simulink library "Control_Signal_Sources"  (R2019b)
settings: Solver=VariableStepAuto  StartTime=0.0  StopTime=10.0  RelTol=1e-3
libraries: simulink x1
settings Model: Creator=mehdi  LastModifiedBy=mehdi

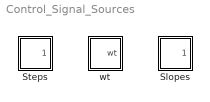
== system Control_Signal_Sources ==
  Slopes : Subsystem  mask(Signal Generator){t=[.2 .4 .6 .8 1  1.2 1.4], v=[7 1 6 2 5 3 4], init_value=0}
      mask prompts: t "Times (s)"; v "Values"; init_value "Init Value"
      mask help: This block made a multi slop ramp signal and used for trigger models during simulation
      mask Display:
      | % t = str2num(get_param(gcb, 't'));
      | % v = str2num(get_param(gcb, 'v'));
      | % [x,y] = stairs(t,v);
      | % plot(x,y)
      | disp('Ramp')
  Steps : Subsystem  mask(Signal Generator){t=[.2 .4 .6 .8 1  1.2 1.4], v=[7 1 6 2 5 3 4]}
      mask prompts: t "Times (s)"; v "Values"
      mask help: This block made a multi level step signal and used for trigger models during simulation
      mask Display:
      | t = str2num(get_param(gcb, 't'));
      | v = str2num(get_param(gcb, 'v'));
      | [x,y] = stairs(t,v);
      | plot(x,y)
  wt : Subsystem  mask(Time Generator){f=100*pi, R=[-pi pi]}
      mask prompts: f "Frequency (rad/s)"; R "Range [min MAX] (rad)"
      mask help: This block generate time for that control block required 'wt'
      mask Display:
      | f=get_param(gcb,'f');
      | f = strjoin(strsplit(f, '*pi'), 'pi');
      | f = strjoin(strsplit(f, 'pi'), '{\\it\\pi}');
      | f = strjoin({f, 't'}, '');
      | disp(f, 'texmode', 'on')

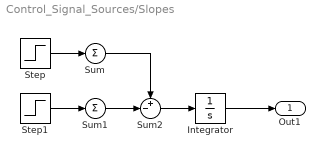
== system Control_Signal_Sources/Slopes ==
  Integrator : Integrator  InitialCondition=init_value
  Step : Step  Time=t  After=v  SampleTime=0
  Step1 : Step  Time=t(2:length(t))  After=v(1:length(v)-1)  SampleTime=0
  Sum : Sum  Inputs=+
  Sum1 : Sum  Inputs=+
  Sum2 : Sum  Inputs=+-|
  Out1 : Outport
  wires:
  Sum1/1 -> Sum2/2
  Step1/1 -> Sum1/1
  Sum/1 -> Sum2/1
  Step/1 -> Sum/1
  Sum2/1 -> Integrator/1
  Integrator/1 -> Out1/1

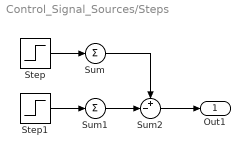
== system Control_Signal_Sources/Steps ==
  Step : Step  Time=t  After=v  SampleTime=0
  Step1 : Step  Time=t(2:length(t))  After=v(1:length(v)-1)  SampleTime=0
  Sum : Sum  Inputs=+
  Sum1 : Sum  Inputs=+
  Sum2 : Sum  Inputs=+-|
  Out1 : Outport
  wires:
  Step/1 -> Sum/1
  Sum/1 -> Sum2/1
  Step1/1 -> Sum1/1
  Sum1/1 -> Sum2/2
  Sum2/1 -> Out1/1

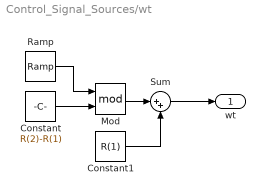
== system Control_Signal_Sources/wt ==
  Constant : Constant  Value=R(2)-R(1)
  Constant1 : Constant  Value=R(1)
  Mod : Math  Operator=mod  SignedPower=off  SaturateOnIntegerOverflow=on
  Ramp : simulink/Sources/Ramp  slope=f  start=0  InitialOutput=0
  Sum : Sum  Inputs=|++
  wt : Outport
  wires:
  Mod/1 -> Sum/1
  Ramp/1 -> Mod/1
  Constant1/1 -> Sum/2
  Sum/1 -> wt/1
  Constant/1 -> Mod/2
